simulink model "modello"  (R2015a)
settings: Solver=ode45  StartTime=0.0  StopTime=20  RelTol=1e-3
undefined symbols (not defined in the file): C, J, Ke, Km, L, M, R, Rd
settings Model: Creator=dell  LastModifiedBy=dell

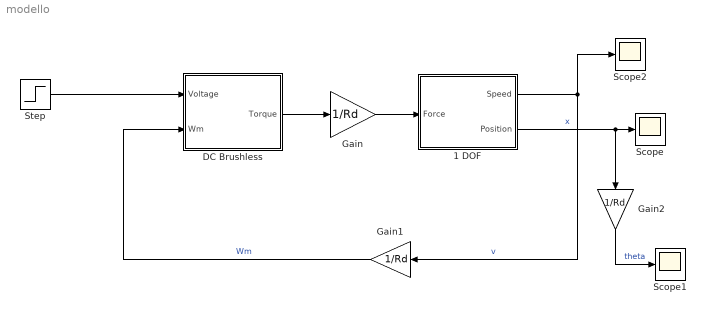
== system modello ==
  "1 DOF " : Subsystem
  DC Brushless : Subsystem
  Gain : Gain  Gain=1/Rd
  Gain1 : Gain  Gain=1/Rd
  Gain2 : Gain  Gain=1/Rd
  Scope : Scope
      settings: TimeRange=20  YMin=1.5e-06  YMax=5.75e-06
  Scope1 : Scope
      settings: TimeRange=20  YMin=0  YMax=0.0015
  Scope2 : Scope
      settings: TimeRange=20  YMin=1.5e-06  YMax=5.75e-06  SaveName=ScopeData3
  Step : Step  After=3.6  SampleTime=0
  wires:
  DC Brushless/1("Torque ") -> Gain/1
  Gain/1 -> "1 DOF "/1(Force)
  Gain1/1 -> DC Brushless/2(Wm)  "Wm"
  Step/1 -> DC Brushless/1("Voltage ")
  "1 DOF "/1("Speed ") -> Gain1/1, Scope2/1  "v"
  "1 DOF "/2("Position ") -> Gain2/1, Scope/1  "x"
  Gain2/1 -> Scope1/1  "theta"

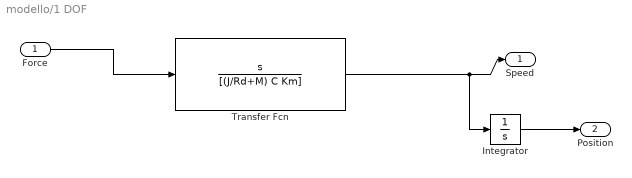
== system modello/1 DOF  ==
  Force : Inport
  Integrator : Integrator
  Transfer Fcn : TransferFcn  Numerator=[1 0]  Denominator=[(J/Rd+M) C Km]
  "Speed " : Outport
  "Position " : Outport  Port=2
  wires:
  Transfer Fcn/1 -> Integrator/1, "Speed "/1
  Force/1 -> Transfer Fcn/1
  Integrator/1 -> "Position "/1

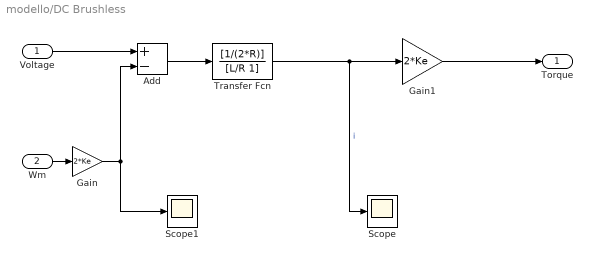
== system modello/DC Brushless ==
  "Voltage " : Inport
  Wm : Inport  Port=2
  Add : Sum  Inputs=+-
  Gain : Gain  Gain=2*Ke
  Gain1 : Gain  Gain=2*Ke
  Scope : Scope
      settings: YMin=-0.075  YMax=0.125  SaveName=ScopeData2
  Scope1 : Scope
      settings: YMin=-0.075  YMax=0.125  SaveName=ScopeData4
  Transfer Fcn : TransferFcn  Numerator=[1/(2*R)]  Denominator=[L/R 1]
  "Torque " : Outport
  wires:
  Gain1/1 -> "Torque "/1
  Transfer Fcn/1 -> Scope/1, Gain1/1  "i"
  Add/1 -> Transfer Fcn/1
  "Voltage "/1 -> Add/1
  Wm/1 -> Gain/1
  Gain/1 -> Scope1/1, Add/2
